simulink library "controller"  (R2020a)
settings: Solver=VariableStepAuto  StartTime=0.0  StopTime=10.0  RelTol=1e-3
values from neighbouring files (symbols this model uses):
  aBooth = block.InputPort(3).Data    [findClosestPointOnPath_sFunc.m]
  bBooth = block.InputPort(4).Data    [findClosestPointOnPath_sFunc.m]
  tau = 0.381966    [BFGS.m]
undefined symbols (not defined in the file or in its folder): kd, ki, kp, meanElev, rDesired
libraries: calc_angle_between_vectors x1, calculate_vector_magnitude x1, filteredPIDController x1, findClosestPointOnPath x1
settings Model: Creator=Ayaz  LastModifiedBy=Ayaz

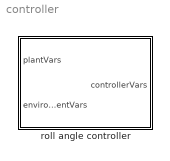
== system controller ==
  roll angle controller : Subsystem  mask{mass=0, pw=0, ph=0, pMeanE=0, rDes=rDesired, kp=kp, ki=ki, kd=kd, tau=tau}
      mask prompts: mass "Kite mass [kg]"; pw "Path width [deg]"; ph "Path height [deg]"; pMeanE "Path mean elevation angle [deg]"; rDes "Desired radius [m]"; kp "Proportional Gain [(m/s)/m]"; ki "Integral Gain [(m/s)/(ms)]"; kd "Derivative Gain [(m/s)/(m/s)]"; tau "Time Constant [s]"
      mask TypeOptions rDes: rDes/Value
      mask TypeOptions kp: filteredPIDController/kp
      mask TypeOptions ki: filteredPIDController/ki
      mask TypeOptions kd: filteredPIDController/kd
      mask TypeOptions tau: filteredPIDController/Value
      mask DialogControl Container3 Prompt: Spooling control

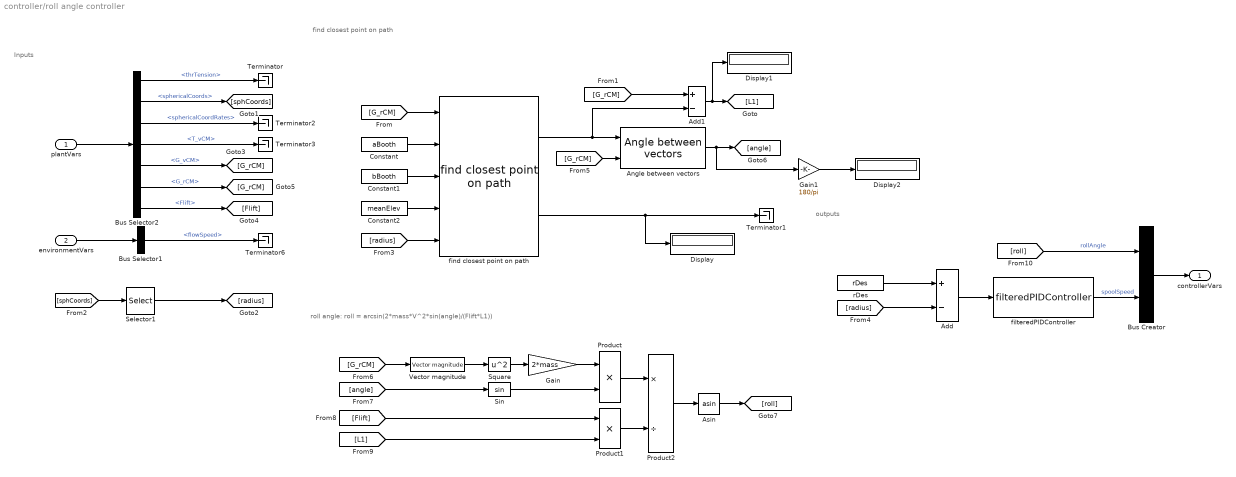
== system controller/roll angle controller ==
  note: find closest point on path
  note: outputs
  note: roll angle: roll = arcsin(2*mass*V^2*sin(angle)/(Flift*L1))
  note: Inputs
  plantVars : Inport
  environmentVars : Inport  Port=2
  Add : Sum  Inputs=+-
  Add1 : Sum  Inputs=+-
  Angle between vectors : calc_angle_between_vectors/Angle between vectors  SystemSampleTime=-1  Latency=0  AutoFrameSizeCalculation=off
  Asin : Trigonometry  Operator=asin
  Bus Creator : BusCreator  Inputs=2
  Bus Selector1 : BusSelector  OutputSignals=flowSpeed
  Bus Selector2 : BusSelector  OutputSignals=thrTension,sphericalCoords,sphericalCoordRates,T_vCM,G_vCM,G_rCM,Flift
  Constant : Constant  Value=aBooth
  Constant1 : Constant  Value=bBooth
  Constant2 : Constant  Value=meanElev
  Display : Display
  Display1 : Display
  Display2 : Display
  Gain : Gain  Gain=2*mass
  Gain1 : Gain  Gain=180/pi
  Product : Product
  Product1 : Product
  Product2 : Product  Inputs=*/
  Selector1 : Selector  InputPortWidth=3  IndexOptions=Index vector (dialog)  Indices=3  OutputSizes=1
  Sin : Trigonometry
  Square : Math  Operator=square  SaturateOnIntegerOverflow=on
  Terminator{,1..3,6} (5 alike) : Terminator
  Vector magnitude : calculate_vector_magnitude/Vector magnitude  SystemSampleTime=-1  Latency=0  AutoFrameSizeCalculation=off
  filteredPIDController : filteredPIDController/filteredPIDController  kp=kp  ki=ki  kd=kd  Value=tau  externalReset=none
  find closest point on path : findClosestPointOnPath/find closest point on path  SystemSampleTime=-1  Latency=0  AutoFrameSizeCalculation=off
      settings: SourceProductBaseCode=SL
  rDes : Constant  Value=rDes
  controllerVars : Outport
  wires:
  plantVars/1 -> Bus Selector2/1
  Bus Selector2/1 -> Terminator/1  "<thrTension>"
  Bus Selector2/2 -> [sphCoords]  "<sphericalCoords>"
  Bus Selector2/3 -> Terminator2/1  "<sphericalCoordRates>"
  Bus Selector2/4 -> Terminator3/1  "<T_vCM>"
  Bus Selector2/5 -> [G_rCM]  "<G_vCM>"
  Bus Selector2/6 -> [G_rCM]  "<G_rCM>"
  Bus Selector1/1 -> Terminator6/1  "<flowSpeed>"
  environmentVars/1 -> Bus Selector1/1
  [roll] -> Bus Creator/1  "rollAngle"
  filteredPIDController/1 -> Bus Creator/2  "spoolSpeed"
  Bus Creator/1 -> controllerVars/1
  [G_rCM] -> find closest point on path/1
  Add/1 -> filteredPIDController/1
  Selector1/1 -> [radius]
  [sphCoords] -> Selector1/1
  [radius] -> find closest point on path/5
  [radius] -> Add/2
  find closest point on path/1 -> Add1/2, Angle between vectors/1
  [G_rCM] -> Add1/1
  [G_rCM] -> Angle between vectors/2
  Add1/1 -> Display1/1, [L1]
  Bus Selector2/7 -> [Flift]  "<Flift>"
  [G_rCM] -> Vector magnitude/1
  Vector magnitude/1 -> Square/1
  Square/1 -> Gain/1
  Gain/1 -> Product/1
  Angle between vectors/1 -> Gain1/1, [angle]
  [angle] -> Sin/1
  Sin/1 -> Product/2
  [Flift] -> Product1/1
  [L1] -> Product1/2
  Product/1 -> Product2/1
  Product1/1 -> Product2/2
  Product2/1 -> Asin/1
  Asin/1 -> [roll]
  find closest point on path/2 -> Display/1, Terminator1/1
  Gain1/1 -> Display2/1
  Constant/1 -> find closest point on path/2
  Constant1/1 -> find closest point on path/3
  Constant2/1 -> find closest point on path/4
  rDes/1 -> Add/1
